simulink library "NeuroMuscularLibrary"  (R2019a)
settings: Solver=ode45  StartTime=0.0  StopTime=10.0  RelTol=1e-3  EnableMultiTasking=on
undefined symbols (not defined in the file): a2loptHAB, a2loptHAD, a2loptHAMsw, a2loptRFsw, ankle_height, aRefHAB, aRefHAD, aRefHAMsw, aRefRFsw, c, c_jointstop, deltaLegAngleThr, DeltaThRef, eref, Fmax, FmaxGLU, footBallToAnkleDist, footBallToCGDist, footBallToCGDist_y, footBallToHeelDist, footCenterlineToBall, footCenterlineToHeel, footInertia, footLength, footMass, FT, FT_GLU, GainDphiHATGLUst, GainDphiHATHABst, GainDphiHATHADst, GainDphiHATHFLst, GainFGASst, GainFGLUst, GainFHABst, GainFHAMst, GainFSOLst, GainFSOLTAst, GainFVASst, GainLBFSHst, GainLBFSHVASst, GainLGLUsw, GainLHABsw, GainLHADsw, GainLHAMGLUsw, GainLHAMsw, GainLRFHFLsw, GainLTAst, GainLTAsw, GainLVASsw, GainPhiHATGLUst, GainPhiHATHABst, GainPhiHATHADst, GainPhiHATHFLst, GainSGLUcHFLst, GainSGLUHAMst, GainSHABcHABst, GainSHADcHADst, GainSHAMBFSHsw, GainSHAMcHFLst, GainSHAMGASsw ... (+175)
libraries: sm_lib x54, $bdroot x45, nesl_utility x39, simulink x24, simulink_extras x6, vrlib x5, dspsigops x4
(part 4 of 5)

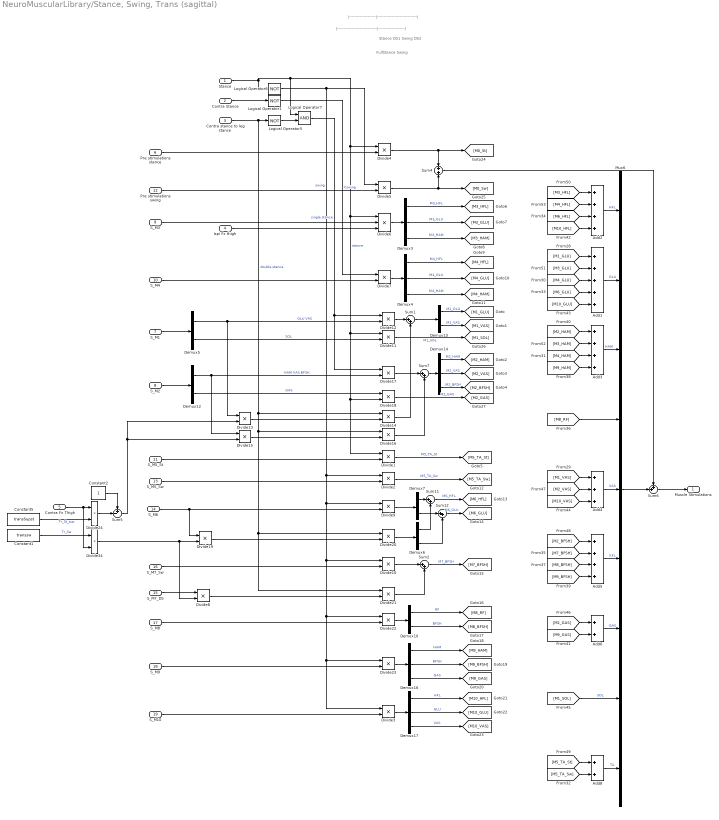
== system NeuroMuscularLibrary/Stance, Swing, Trans (sagittal) ==
  note: Stance DS1 Swing DS2
  note: FullStance Swing
  note: |------------------------------|--------------------|
  note: |--------------------|------------------------------|
  Stance : Inport
  Contra Stance : Inport  Port=2
  Contra stance to leg stance : Inport  Port=3
  Ispi Fx thigh : Inport  Port=4
  Contra Fx Thigh : Inport  Port=5
  Pre stimulations stance : Inport  Port=6
  S_M1 : Inport  Port=7
  S_M2 : Inport  Port=8
  S_M3 : Inport  Port=9
  S_M4 : Inport  Port=10
  S_M5_St : Inport  Port=11
  Pre stimulations swing : Inport  Port=12
  S_M5_Sw : Inport  Port=13
  S_M6 : Inport  Port=14
  S_M7_DS : Inport  Port=15
  S_M7_Sw : Inport  Port=16
  S_M8 : Inport  Port=17
  S_M9 : Inport  Port=18
  S_M10 : Inport  Port=19
  Add1 : Sum  Inputs=5
  Add2 : Sum  Inputs=4
  Add3 : Sum  Inputs=4
  Add4 : Sum  Inputs=3
  Add5 : Sum  Inputs=4
  Add6 : Sum  Inputs=2
  Add8 : Sum  Inputs=2
  Constant1 : Constant  Value=transsw
  Constant2 : Constant
  Constant5 : Constant  Value=transSupst
  Demux{6..7,10,13} (4 alike) : Demux  Outputs=2
  Demux12 : Demux  Outputs=[3 1]
  Demux{3..4,14,16..17} (5 alike) : Demux  Outputs=3
  Demux5 : Demux  Outputs=[2 1]
  Divide{1..5,7..24,34} (24 alike) : Product
  Divide6 : Product  Inputs=3
  Logical Operator1 : Logic  Operator=NOT  AllPortsSameDT=off  OutDataTypeStr=boolean
  Logical Operator5 : Logic  Operator=NOT  AllPortsSameDT=off  OutDataTypeStr=boolean
  Logical Operator6 : Logic  Operator=NOT  AllPortsSameDT=off  OutDataTypeStr=boolean
  Logical Operator7 : Logic  AllPortsSameDT=off  OutDataTypeStr=boolean
  Mux6 : Mux  Inputs=9
  Sum{1..2,7,11..12} (5 alike) : Sum  Inputs=|++  SaturateOnIntegerOverflow=on  InputSameDT=on  OutDataTypeStr=Inherit: Same as first input
  Sum4 : Sum  SaturateOnIntegerOverflow=on  InputSameDT=on  OutDataTypeStr=Inherit: Same as first input
  Sum5 : Sum  Inputs=+-|  SaturateOnIntegerOverflow=on  InputSameDT=on  OutDataTypeStr=Inherit: Same as first input
  Sum6 : Sum  Inputs=++|  SaturateOnIntegerOverflow=on  InputSameDT=on  OutDataTypeStr=Inherit: Same as first input
  Muscle Stimulations : Outport  OutputWhenDisabled=reset  InitialOutput=0  VectorParamsAs1DForOutWhenUnconnected=on
  wires:
  Stance/1 -> Logical Operator7/1, Divide4/1, Divide11/1, Divide18/2, Divide1/1, Divide6/1, Logical Operator6/1  "stance"
  Contra stance to leg stance/1 -> Logical Operator5/1, Divide14/1, Divide16/1, Divide20/1, Divide21/1  "double stance"
  Logical Operator5/1 -> Logical Operator7/2
  S_M4/1 -> Divide7/2
  Contra Stance/1 -> Logical Operator1/1
  Logical Operator1/1 -> Divide7/1  "Cswing"
  Constant5/1 -> Divide24/2  "Tr_St_sup"
  Divide24/1 -> Sum5/2
  Constant2/1 -> Sum5/1
  Contra Fx Thigh/1 -> Divide24/1, Divide34/2
  Demux4/1 -> [M4_HFL]  "M4_HFL"
  Add2/1 -> Mux6/1  "HFL"
  Add1/1 -> Mux6/2  "GLU"
  Demux4/2 -> [M4_GLU]  "M4_GLU"
  Add3/1 -> Mux6/3  "HAM"
  Demux4/3 -> [M4_HAM]  "M4_HAM"
  Add4/1 -> Mux6/5  "VAS"
  Add5/1 -> Mux6/6  "KFL"
  Add6/1 -> Mux6/7  "GAS"
  Add8/1 -> Mux6/9  "TA"
  Constant1/1 -> Divide34/1  "Tr_Sw"
  Divide7/1 -> Demux4/1
  Logical Operator7/1 -> Divide12/1, Divide17/1  "single stance"
  Divide34/1 -> Divide19/2, Divide8/2
  Logical Operator6/1 -> Divide5/1, Divide2/1, Divide9/1, Divide10/1, Divide3/1, Divide23/1, Divide22/1  "swing"
  Mux6/1 -> Sum6/2
  Sum6/1 -> Muscle Stimulations/1
  Sum4/1 -> Sum6/1
  Pre stimulations swing/1 -> Divide5/2
  Pre stimulations stance/1 -> Divide4/2
  Divide5/1 -> [M0_Sw], Sum4/2
  Divide4/1 -> Sum4/1, [M0_St]
  S_M1/1 -> Demux5/1
  S_M2/1 -> Demux12/1
  Demux5/1 -> Divide12/2, Divide13/1  "GLU VAS"
  Demux5/2 -> Divide11/2  "SOL"
  Divide12/1 -> Sum1/1
  Divide13/1 -> Divide14/2
  Divide14/1 -> Sum1/2
  Divide16/1 -> Sum7/2
  Divide15/1 -> Divide16/2
  Sum1/1 -> Demux13/1
  Demux13/1 -> [M1_GLU]  "M1_GLU"
  Demux13/2 -> [M1_VAS]  "M1_VAS"
  Demux12/1 -> Divide17/2, Divide15/1  "HAM VAS BFSH"
  Divide17/1 -> Sum7/1
  Sum7/1 -> Demux14/1
  Demux14/1 -> [M2_HAM]  "M2_HAM"
  Demux14/2 -> [M2_VAS]  "M2_VAS"
  Demux14/3 -> [M2_BFSH]  "M2_BFSH"
  Demux12/2 -> Divide18/1  "GAS"
  Divide18/1 -> [M2_GAS]  "M2_GAS"
  S_M5_St/1 -> Divide1/2
  Divide1/1 -> [M5_TA_St]  "M5_TA_St"
  Divide11/1 -> [M1_SOL]  "M1_SOL"
  S_M3/1 -> Divide6/2
  Ispi Fx thigh/1 -> Divide6/3
  Divide6/1 -> Demux3/1
  Demux3/1 -> [M3_HFL]  "M3_HFL"
  Demux3/2 -> [M3_GLU]  "M3_GLU"
  Demux3/3 -> [M3_HAM]  "M3_HAM"
  S_M5_Sw/1 -> Divide2/2
  Divide2/1 -> [M5_TA_Sw]  "M5_TA_Sw"
  S_M6/1 -> Divide9/2, Divide19/1
  Divide9/1 -> Demux7/1
  Demux7/2 -> Sum12/1
  Divide20/1 -> Demux6/1
  Demux6/1 -> Sum11/2
  Demux6/2 -> Sum12/2
  Demux7/1 -> Sum11/1
  Divide19/1 -> Divide20/2
  Sum11/1 -> [M6_HFL]  "M6_HFL"
  Sum12/1 -> [M6_GLU]  "M6_GLU"
  Divide10/1 -> Sum2/1
  Divide21/1 -> Sum2/2
  Sum5/1 -> Divide13/2, Divide15/2
  S_M7_Sw/1 -> Divide10/2
  Divide8/1 -> Divide21/2
  S_M7_DS/1 -> Divide8/1
  Sum2/1 -> [M7_BFSH]  "M7_BFSH"
  S_M8/1 -> Divide22/2
  Divide22/1 -> Demux10/1
  S_M9/1 -> Divide23/2
  Divide23/1 -> Demux16/1
  S_M10/1 -> Divide3/2
  Divide3/1 -> Demux17/1
  Demux10/2 -> [M8_BFSH]  "BFSH"
  Demux10/1 -> [M8_RF]  "RF"
  Demux16/1 -> [M9_HAM]  "HAM"
  Demux16/2 -> [M9_BFSH]  "BFSH"
  Demux16/3 -> [M9_GAS]  "GAS"
  Demux17/1 -> [M10_HFL]  "HFL"
  Demux17/2 -> [M10_GLU]  "GLU"
  Demux17/3 -> [M10_VAS]  "VAS"
  [M1_GLU] -> Add1/1
  [M3_GLU] -> Add1/2
  [M4_GLU] -> Add1/3
  [M6_GLU] -> Add1/4
  [M10_GLU] -> Add1/5
  [M1_VAS] -> Add4/1
  [M2_HAM] -> Add3/1
  [M2_VAS] -> Add4/2
  [M2_BFSH] -> Add5/1
  [M2_GAS] -> Add6/1
  [M3_HFL] -> Add2/1
  [M3_HAM] -> Add3/2
  [M4_HFL] -> Add2/2
  [M4_HAM] -> Add3/3
  [M5_TA_St] -> Add8/1
  [M5_TA_Sw] -> Add8/2
  [M6_HFL] -> Add2/3
  [M7_BFSH] -> Add5/2
  [M9_BFSH] -> Add5/4
  [M8_BFSH] -> Add5/3
  [M8_RF] -> Mux6/4
  [M9_HAM] -> Add3/4
  [M9_GAS] -> Add6/2
  [M10_HFL] -> Add2/4
  [M10_VAS] -> Add4/3
  [M1_SOL] -> Mux6/8  "SOL"

== system NeuroMuscularLibrary/Swing Phase (coronal) ==
  note: Swing Phase Control
  note: M6: swing hip
  Target Angle Coronal : Inport
  LceHAD : Inport  Port=2
  LceHAB : Inport  Port=3
  Enable : EnablePort  StatesWhenEnabling=reset  ZeroCross=off
  " 1" : Gain  Gain=a2loptHAB
  " 2" : Gain  Gain=a2loptHAD
  " 3" : Gain  Gain=GainLHABsw
  " 4" : Gain  Gain=GainLHADsw
  Constant1 : Constant
  Constant12 : Constant  Value=PreStimHADsw
  Constant15 : Constant  Value=PreStimHABsw
  Constant2 : Constant  Value=aRefHAB
  Constant3 : Constant  Value=aRefHAD
  Constant5 : Constant
  Mux : Mux  Inputs=2
  Mux1 : Mux  Inputs=2
  Sum1 : Sum  Inputs=-+|  SaturateOnIntegerOverflow=on  InputSameDT=on  OutDataTypeStr=Inherit: Same as first input
  Sum10 : Sum  Inputs=++|  SaturateOnIntegerOverflow=on  InputSameDT=on  OutDataTypeStr=Inherit: Same as first input
  Sum13 : Sum  Inputs=|-+  SaturateOnIntegerOverflow=on  InputSameDT=on  OutDataTypeStr=Inherit: Same as first input
  Sum2 : Sum  Inputs=-+|  SaturateOnIntegerOverflow=on  InputSameDT=on  OutDataTypeStr=Inherit: Same as first input
  Sum3 : Sum  Inputs=+-|  SaturateOnIntegerOverflow=on  InputSameDT=on  OutDataTypeStr=Inherit: Same as first input
  Sum4 : Sum  Inputs=+-|  SaturateOnIntegerOverflow=on  InputSameDT=on  OutDataTypeStr=Inherit: Same as first input
  positive half1 : Saturate  UpperLimit=inf  LowerLimit=0  ZeroCross=off
  positive half2 : Saturate  UpperLimit=inf  LowerLimit=0  ZeroCross=off
  S_0_Sw : Outport  OutputWhenDisabled=reset  InitialOutput=0  VectorParamsAs1DForOutWhenUnconnected=on
  S_M6 [HAB HAD] : Outport  Port=2  OutputWhenDisabled=reset  InitialOutput=0  VectorParamsAs1DForOutWhenUnconnected=on
  wires:
  Mux/1 -> S_0_Sw/1
  Constant5/1 -> Sum10/1
  Sum13/1 -> " 1"/1
  " 1"/1 -> Sum10/2
  Sum10/1 -> Sum1/1  "lceOffHAB"
  Sum1/1 -> positive half2/1
  positive half2/1 -> " 3"/1
  Constant1/1 -> Sum3/1
  Target Angle Coronal/1 -> Sum13/2, Sum4/1
  Sum4/1 -> " 2"/1
  " 2"/1 -> Sum3/2
  Sum3/1 -> Sum2/1  "lceOffHAD"
  Sum2/1 -> positive half1/1
  positive half1/1 -> " 4"/1
  LceHAB/1 -> Sum1/2
  LceHAD/1 -> Sum2/2
  " 3"/1 -> Mux1/1  "HAB"
  " 4"/1 -> Mux1/2  "HAD"
  Mux1/1 -> S_M6 [HAB HAD]/1
  Constant15/1 -> Mux/1
  Constant12/1 -> Mux/2
  Constant2/1 -> Sum13/1
  Constant3/1 -> Sum4/2

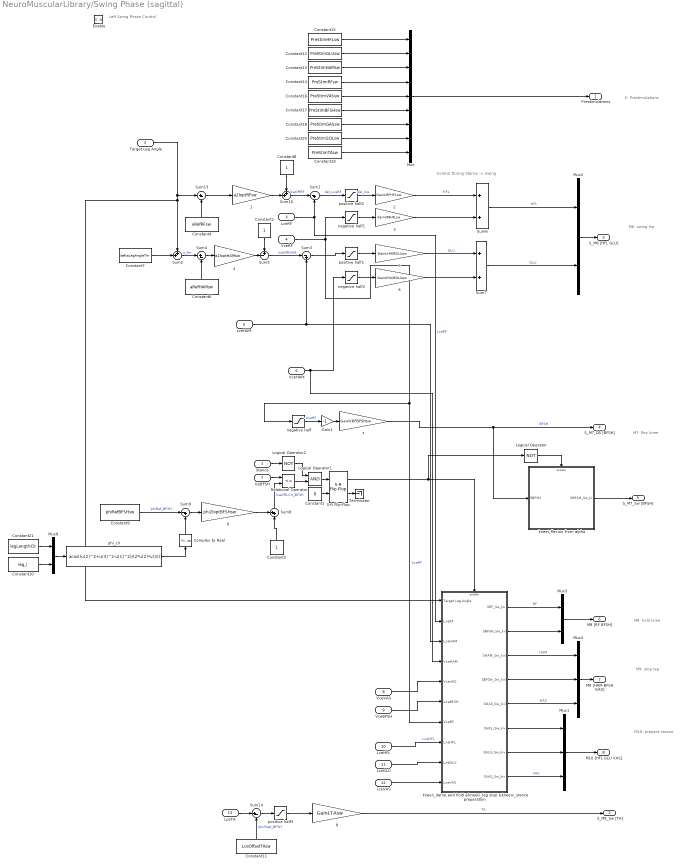
== system NeuroMuscularLibrary/Swing Phase (sagittal) ==
  note: Left Swing Phase Control
  note: Control During Stance -> Swing
  note: 0: Prestimulations
  note: M6: swing hip
  note: M7: flex knee
  note: M8: hold knee
  note: M9: stop leg
  note: M10: prepare stance
  Stance : Inport
  "Target Leg Angle " : Inport  Port=2
  LceRF : Inport  Port=3
  VceRF : Inport  Port=4
  LceHAM : Inport  Port=5
  VceHAM : Inport  Port=6
  lceBFSH : Inport  Port=7
  VceVAS : Inport  Port=8
  VceBFSH : Inport  Port=9
  LceHFL : Inport  Port=10
  LceGLU : Inport  Port=11
  LceVAS : Inport  Port=12
  LceTA : Inport  Port=13
  Enable : EnablePort  StatesWhenEnabling=reset  ZeroCross=off
  " 1" : Gain  Gain=a2loptRFsw
  " 2" : Gain  Gain=GainLRFHFLsw
  " 3" : Gain  Gain=GainVRFHFLsw
  " 4" : Gain  Gain=a2loptHAMsw
  " 5" : Gain  Gain=GainLHAMGLUsw
  " 6" : Gain  Gain=GainVHAMGLUsw
  " 7" : Gain  Gain=GainVRFBFSHsw
  " 8" : Gain  Gain=GainLTAsw
  " 9" : Gain  Gain=phi2loptBFSHsw
  Complex to Real : ComplexToRealImag  Output=Real
  Constant1 : Constant  Value=0  OutDataTypeStr=boolean
  Constant10 : Constant  Value=leg_l
  Constant11 : Constant  Value=LceOffsetTAsw
  Constant12 : Constant  Value=PreStimGLUsw
  Constant13 : Constant  Value=PreStimHAMsw
  Constant14 : Constant  Value=PreStimRFsw
  Constant15 : Constant  Value=PreStimHFLsw
  Constant16 : Constant  Value=PreStimVASsw
  Constant17 : Constant  Value=PreStimBFSHsw
  Constant18 : Constant  Value=PreStimGASsw
  Constant19 : Constant  Value=PreStimTAsw
  Constant2 : Constant
  Constant20 : Constant  Value=PreStimSOLsw
  Constant21 : Constant  Value=legLengthClr
  Constant3 : Constant
  Constant4 : Constant  Value=aRefRFsw
  Constant6 : Constant  Value=aRefHAMsw
  Constant7 : Constant  Value=deltaLegAngleThr
  Constant8 : Constant
  Constant9 : Constant  Value=phiRefBFSHsw
  Gain1 : Gain  Gain=-1
  Logical Operator : Logic  Operator=NOT  AllPortsSameDT=off  OutDataTypeStr=boolean
  Logical Operator1 : Logic  AllPortsSameDT=off  OutDataTypeStr=boolean
  Logical Operator2 : Logic  Operator=NOT  AllPortsSameDT=off  OutDataTypeStr=boolean
  Mux : Mux  Inputs=9
  Mux1 : Mux  Inputs=3
  Mux2 : Mux  Inputs=2
  Mux3 : Mux  Inputs=2
  Mux4 : Mux  Inputs=3
  Mux8 : Mux  Inputs=2
  Relational Operator : RelationalOperator  Operator=<=  OutDataTypeStr=boolean  ZeroCross=off  RndMeth=Nearest
  S-R Flip-Flop : simulink_extras/Flip Flops/S-R Flip-Flop  initial_condition=0
  Sum1 : Sum  Inputs=|-+  SaturateOnIntegerOverflow=on  InputSameDT=on  OutDataTypeStr=Inherit: Same as first input
  Sum10 : Sum  Inputs=++|  SaturateOnIntegerOverflow=on  InputSameDT=on  OutDataTypeStr=Inherit: Same as first input
  Sum13 : Sum  Inputs=|+-  SaturateOnIntegerOverflow=on  InputSameDT=on  OutDataTypeStr=Inherit: Same as first input
  Sum14 : Sum  Inputs=|+-  SaturateOnIntegerOverflow=on  InputSameDT=on  OutDataTypeStr=Inherit: Same as first input
  Sum2 : Sum  Inputs=++|  SaturateOnIntegerOverflow=on  InputSameDT=on  OutDataTypeStr=Inherit: Same as first input
  Sum3 : Sum  Inputs=|-+  SaturateOnIntegerOverflow=on  InputSameDT=on  OutDataTypeStr=Inherit: Same as first input
  Sum4 : Sum  Inputs=|+-  SaturateOnIntegerOverflow=on  InputSameDT=on  OutDataTypeStr=Inherit: Same as first input
  Sum5 : Sum  Inputs=+-|  SaturateOnIntegerOverflow=on  InputSameDT=on  OutDataTypeStr=Inherit: Same as first input
  Sum6 : Sum  SaturateOnIntegerOverflow=on  InputSameDT=on  OutDataTypeStr=Inherit: Same as first input
  Sum7 : Sum  SaturateOnIntegerOverflow=on  InputSameDT=on  OutDataTypeStr=Inherit: Same as first input
  Sum8 : Sum  Inputs=++|  SaturateOnIntegerOverflow=on  InputSameDT=on  OutDataTypeStr=Inherit: Same as first input
  Sum9 : Sum  Inputs=|-+  SaturateOnIntegerOverflow=on  InputSameDT=on  OutDataTypeStr=Inherit: Same as first input
  Terminator : Terminator
  kneei_flexion from alpha : Subsystem  TreatAsAtomicUnit=on
  kneeii_damp and hold &kneeiii_leg stop &kneeiv_stance preparation : Subsystem  TreatAsAtomicUnit=on
  negative half : Saturate  UpperLimit=0  LowerLimit=-inf  ZeroCross=off
  negative half1 : Saturate  UpperLimit=0  LowerLimit=-inf  ZeroCross=off
  negative half2 : Saturate  UpperLimit=0  LowerLimit=-inf  ZeroCross=off
  phi_clr : Fcn  Expr=acos((u(2)^2+u(3)^2-u(1)^2)/(2*u(2)*u(3)))
  positive half1 : Saturate  UpperLimit=inf  LowerLimit=0  ZeroCross=off
  positive half2 : Saturate  UpperLimit=inf  LowerLimit=0  ZeroCross=off
  positive half3 : Saturate  UpperLimit=inf  LowerLimit=0  ZeroCross=off
  Prestimulations : Outport  OutputWhenDisabled=reset  InitialOutput=0  VectorParamsAs1DForOutWhenUnconnected=on
  S_M5_Sw [TA] : Outport  Port=2  OutputWhenDisabled=reset  InitialOutput=0  VectorParamsAs1DForOutWhenUnconnected=on
  S_M6 [HFL GLU] : Outport  Port=3  OutputWhenDisabled=reset  InitialOutput=0  VectorParamsAs1DForOutWhenUnconnected=on
  S_M7_DS [BFSH] : Outport  Port=4  OutputWhenDisabled=reset  InitialOutput=0  VectorParamsAs1DForOutWhenUnconnected=on
  S_M7_Sw [BFSH] : Outport  Port=5  OutputWhenDisabled=reset  InitialOutput=0  VectorParamsAs1DForOutWhenUnconnected=on
  M8 [RF BFSH] : Outport  Port=6  OutputWhenDisabled=reset  InitialOutput=0  VectorParamsAs1DForOutWhenUnconnected=on
  M9 [HAM BFSH GAS] : Outport  Port=7  OutputWhenDisabled=reset  InitialOutput=0  VectorParamsAs1DForOutWhenUnconnected=on
  M10 [HFL GLU VAS] : Outport  Port=8  OutputWhenDisabled=reset  InitialOutput=0  VectorParamsAs1DForOutWhenUnconnected=on
  wires:
  "Target Leg Angle "/1 -> kneeii_damp and hold &kneeiii_leg stop &kneeiv_stance preparation/1(Target Leg Angle), Sum2/1, Sum13/1
  Sum13/1 -> " 1"/1
  " 1"/1 -> Sum10/2
  Sum1/1 -> positive half2/1  "del_LceRF"
  positive half2/1 -> " 2"/1  "del_lce"
  Sum2/1 -> Sum4/1  "a_thr"
  Constant2/1 -> Sum5/1
  " 4"/1 -> Sum5/2
  Sum3/1 -> positive half1/1
  positive half1/1 -> " 5"/1
  Sum5/1 -> Sum3/1  "lceOffHAM"
  LceHAM/1 -> Sum3/2, kneeii_damp and hold &kneeiii_leg stop &kneeiv_stance preparation/3(LceHAM)
  Gain1/1 -> " 7"/1
  negative half/1 -> Gain1/1  "-VceRF"
  " 7"/1 -> kneei_flexion from alpha/1(SBFSH), S_M7_DS [BFSH]/1  "BFSH"
  Constant1/1 -> S-R Flip-Flop/2
  S-R Flip-Flop/2 -> Terminator/1
  S-R Flip-Flop/1 -> Logical Operator/1, kneeii_damp and hold &kneeiii_leg stop &kneeiv_stance preparation/Enable
  Logical Operator/1 -> kneei_flexion from alpha/Enable
  lceBFSH/1 -> Relational Operator/1
  Mux8/1 -> phi_clr/1
  Constant21/1 -> Mux8/1
  Constant10/1 -> Mux8/2
  Sum9/1 -> " 9"/1
  Constant9/1 -> Sum9/1  "phiRef_BFSH"
  phi_clr/1 -> Complex to Real/1
  Constant3/1 -> Sum8/2
  " 9"/1 -> Sum8/1
  Sum8/1 -> Relational Operator/2  "lceOffLClr_BFSH"
  VceBFSH/1 -> kneeii_damp and hold &kneeiii_leg stop &kneeiv_stance preparation/6(VceBFSH)
  LceHFL/1 -> kneeii_damp and hold &kneeiii_leg stop &kneeiv_stance preparation/8(LceHFL)  "LceHFL"
  LceGLU/1 -> kneeii_damp and hold &kneeiii_leg stop &kneeiv_stance preparation/9(LceGLU)
  LceVAS/1 -> kneeii_damp and hold &kneeiii_leg stop &kneeiv_stance preparation/10(LceVAS)
  kneeii_damp and hold &kneeiii_leg stop &kneeiv_stance preparation/6(SHFL_Sw_kiv) -> Mux1/1
  kneeii_damp and hold &kneeiii_leg stop &kneeiv_stance preparation/7(SGLU_Sw_kiv) -> Mux1/2
  kneei_flexion from alpha/1(SBFSH_Sw_ki) -> S_M7_Sw [BFSH]/1
  kneeii_damp and hold &kneeiii_leg stop &kneeiv_stance preparation/2(SBFSH_Sw_kii) -> Mux3/2
  kneeii_damp and hold &kneeiii_leg stop &kneeiv_stance preparation/4(SBFSH_Sw_kiii) -> Mux4/2
  Sum14/1 -> positive half3/1
  LceTA/1 -> Sum14/1
  positive half3/1 -> " 8"/1
  Logical Operator1/1 -> S-R Flip-Flop/1
  Relational Operator/1 -> Logical Operator1/2
  Stance/1 -> Logical Operator2/1
  Logical Operator2/1 -> Logical Operator1/1
  kneeii_damp and hold &kneeiii_leg stop &kneeiv_stance preparation/3(SHAM_Sw_kiii) -> Mux4/1  "HAM"
  kneeii_damp and hold &kneeiii_leg stop &kneeiv_stance preparation/1(SRF_Sw_kii) -> Mux3/1  "RF"
  kneeii_damp and hold &kneeiii_leg stop &kneeiv_stance preparation/8(SVAS_Sw_kiv) -> Mux1/3  "VAS"
  " 8"/1 -> S_M5_Sw [TA]/1  "TA"
  kneeii_damp and hold &kneeiii_leg stop &kneeiv_stance preparation/5(SGAS_Sw_kiii) -> Mux4/3  "GAS"
  Mux2/1 -> S_M6 [HFL GLU]/1
  Mux3/1 -> M8 [RF BFSH]/1
  Mux4/1 -> M9 [HAM BFSH GAS]/1
  Mux1/1 -> M10 [HFL GLU VAS]/1
  LceRF/1 -> kneeii_damp and hold &kneeiii_leg stop &kneeiv_stance preparation/2(LceRF), Sum1/2  "LceRF"
  VceVAS/1 -> kneeii_damp and hold &kneeiii_leg stop &kneeiv_stance preparation/5(VceVAS)
  VceRF/1 -> kneeii_damp and hold &kneeiii_leg stop &kneeiv_stance preparation/7(VceRF), negative half/1, negative half1/1  "VceRF"
  VceHAM/1 -> kneeii_damp and hold &kneeiii_leg stop &kneeiv_stance preparation/4(VceHAM), negative half2/1
  " 2"/1 -> Sum6/1  "HFL"
  " 3"/1 -> Sum6/2
  Sum6/1 -> Mux2/1  "HFL"
  negative half1/1 -> " 3"/1
  negative half2/1 -> " 6"/1
  " 5"/1 -> Sum7/1  "GLU"
  Sum7/1 -> Mux2/2  "GLU"
  " 6"/1 -> Sum7/2
  Constant4/1 -> Sum13/2
  Constant7/1 -> Sum2/2
  Constant6/1 -> Sum4/2
  Constant8/1 -> Sum10/1
  Sum10/1 -> Sum1/1  "lceOffRF"
  Sum4/1 -> " 4"/1
  Constant11/1 -> Sum14/2  "phi2lopt_BFSH"
  Constant14/1 -> Mux/4
  Constant12/1 -> Mux/2
  Mux/1 -> Prestimulations/1
  Constant19/1 -> Mux/9
  Constant17/1 -> Mux/6
  Constant18/1 -> Mux/7
  Constant15/1 -> Mux/1
  Constant13/1 -> Mux/3
  Constant16/1 -> Mux/5
  Constant20/1 -> Mux/8
  Complex to Real/1 -> Sum9/2

== system NeuroMuscularLibrary/TA Link ==
  note: TA Attachment
  Ankle angle  [rad] : Inport
  Constant : Constant  Value=lslackTA+loptTA
  Constant3 : Constant  Value=phimaxTA
  Constant5 : Constant  Value=phirefTA
  Demux1 : Demux  Outputs=2
  Gain2 : Gain  Gain=rTAmax
  Gain3 : Gain  Gain=phiScaleTA
  Gain8 : Gain  Gain=phiScaleTA
  Gain9 : Gain  Gain=rhoTA/phiScaleTA
  Mux1 : Mux  Inputs=2
  Sum4 : Sum  Inputs=-+
  Sum5 : Sum  Inputs=|++
  Sum6 : Sum  Inputs=|+-
  Sum7 : Sum  Inputs=-+|
  length change term : Trigonometry
  offset correction term : Trigonometry
  variable lever term : Trigonometry  Operator=cos
  lmtc [m] : Outport  VectorParamsAs1DForOutWhenUnconnected=on
  lever [m] : Outport  Port=2  VectorParamsAs1DForOutWhenUnconnected=on
  wires:
  Sum7/1 -> Gain3/1
  Sum6/1 -> Gain8/1
  length change term/1 -> Sum4/2
  variable lever term/1 -> Mux1/2
  Gain8/1 -> offset correction term/1
  Sum4/1 -> Mux1/1
  Constant5/1 -> Sum6/1
  Mux1/1 -> Gain2/1
  Gain9/1 -> Sum5/2
  Demux1/2 -> lever [m]/1
  Sum5/1 -> lmtc [m]/1
  Constant3/1 -> Sum7/1, Sum6/2
  offset correction term/1 -> Sum4/1
  Gain3/1 -> variable lever term/1, length change term/1
  Gain2/1 -> Demux1/1
  Demux1/1 -> Gain9/1
  Constant/1 -> Sum5/1
  Ankle angle  [rad]/1 -> Sum7/2

== system NeuroMuscularLibrary/Target leg angle calculator ==
  note: positive for left, negative for right
  Saggital d,v : Inport
  Coronal d,v : Inport  Port=2
  HATy : Inport  Port=3
  HATyInt : Inport  Port=4
  " 1" : Gain  Gain=simbiconGainV
  " 2" : Gain  Gain=simbiconGainV_C
  " 3" : Gain  Gain=simbiconGainD
  " 4" : Gain  Gain=simbiconGainD_C
  " 5" : Gain  Gain=headingGain
  " 6" : Gain  Gain=headingIntGain
  Add : Sum  Inputs=+--
  Add1 : Sum  Inputs=+++++
  Constant2 : Constant  Value=simbiconLegAngle0
  Constant7 : Constant  Value=simbiconLegAngle0_C
  Demux : Demux  Outputs=2
  Demux1 : Demux  Outputs=2
  "Saggital Target leg angle " : Outport  VectorParamsAs1DForOutWhenUnconnected=on
  "Coronal Target leg angle " : Outport  Port=2  VectorParamsAs1DForOutWhenUnconnected=on
  wires:
  Saggital d,v/1 -> Demux/1
  Coronal d,v/1 -> Demux1/1
  Demux/1 -> " 3"/1  "d"
  Demux/2 -> " 1"/1  "v"
  Demux1/1 -> " 4"/1  "d"
  Demux1/2 -> " 2"/1  "v"
  " 1"/1 -> Add/3
  " 3"/1 -> Add/2
  Constant2/1 -> Add/1
  Constant7/1 -> Add1/1
  " 4"/1 -> Add1/2
  " 2"/1 -> Add1/3
  Add/1 -> "Saggital Target leg angle "/1
  HATy/1 -> " 5"/1
  " 5"/1 -> Add1/4
  Add1/1 -> "Coronal Target leg angle "/1
  " 6"/1 -> Add1/5
  HATyInt/1 -> " 6"/1

== system NeuroMuscularLibrary/Thigh Sensor Sheet ==
  note: Inner Segment Pressure Sheet
  Gain3 : Gain  Gain=k_pressure
  Gain4 : Gain  Gain=1/v_max_pressure
  Mux1 : Mux  Inputs=2
  PS-Simulink Converter : nesl_utility/PS-Simulink Converter  PhysicalDomain=network_engine_domain  SubClassName=ps_output  LeftPortType=input  RightPortType=output  PseudoPeriodic=off  Frequencies=[]  Unit=m/s  AffineConversion=off
  PS-Simulink Converter1 : nesl_utility/PS-Simulink Converter  PhysicalDomain=network_engine_domain  SubClassName=ps_output  LeftPortType=input  RightPortType=output  PseudoPeriodic=off  Frequencies=[]  Unit=m  AffineConversion=off
  Pressure Sheet Reaction Force : Fcn  Expr=-u(1) * (1+sgn(u(1))*u(2))
  Prismatic Joint : sm_lib/Joints/Prismatic Joint  SenseConstraintForce=off  SenseConstraintForceX=off  SenseConstraintForceY=off  SenseConstraintForceZ=off  SenseConstraintTorque=off  SenseConstraintTorqueX=off  SenseConstraintTorqueY=off  SenseConstraintTorqueZ=off  SenseTotalForce=off  SenseTotalForceX=off  SenseTotalForceY=off  SenseTotalForceZ=off  SenseTotalTorque=off  SenseTotalTorqueX=off  SenseTotalTorqueY=off  SenseTotalTorqueZ=off  CompositeWrenchDir=FollowerOnBase  CompositeWrenchFrame=BaseFrame  EquilibriumPosition=0  EquilibriumPositionUnits=m  SpringStiffness=0  SpringStiffnessUnits=N/m  DampingCoefficient=0  DampingCoefficientUnits=N/(m/s)  TorqueActuationMode=InputTorque  MotionActuationMode=ComputedMotion  SensePosition=on  SenseVelocity=on  SenseAcceleration=off  SenseTorqueForce=off  SenseLowerLimitTorqueForce=off  SenseUpperLimitTorqueForce=off  LowerLimitSpecify=off  LowerLimitBound=-1  LowerLimitBoundUnits=m  LowerLimitStiffness=1e6  LowerLimitStiffnessUnits=N/m  LowerLimitDamping=1e3  LowerLimitDampingUnits=N/(m/s)  LowerLimitTransitionRegionWidth=1e-4  LowerLimitTransitionRegionWidthUnits=m  UpperLimitSpecify=off  UpperLimitBound=1  UpperLimitBoundUnits=m  UpperLimitStiffness=1e6  UpperLimitStiffnessUnits=N/m  UpperLimitDamping=1e3  UpperLimitDampingUnits=N/(m/s)  UpperLimitTransitionRegionWidth=1e-4  UpperLimitTransitionRegionWidthUnits=m  PositionTargetSpecify=on  PositionTargetPriority=High  PositionTargetValue=0  PositionTargetValueUnits=m  VelocityTargetSpecify=on  VelocityTargetPriority=High  VelocityTargetValue=0  VelocityTargetValueUnits=m/s
  Rigid Transform : sm_lib/Frames and Transforms/Rigid Transform  TranslationMethod=None  TranslationStandardOffset=0  TranslationLengthUnit=m  TranslationStandardAxis=+Z  TranslationCartesianOffset=[0 0 0]  TranslationROffset=0  TranslationROffsetUnits=m  TranslationZOffset=0  TranslationZOffsetUnits=m  TranslationThetaOffset=0  TranslationThetaOffsetUnits=deg  RotationMethod=AlignedAxes  RotationAngleUnits=deg  RotationStandardAxis=+Z  RotationAngle=0.0  RotationArbitraryAxis=[0 0 1]  FollAlignAxisA=+Z  BaseAlignAxisA=+X  FollAlignAxisB=+Y  BaseAlignAxisB=+Y  RotationSequenceAxes=FollowerAxes  RotationSequence=XYX  RotationSequenceAngles=[0 0 0]  RotationSequenceAnglesUnits=deg  RotationMatrix=[1 0 0; 0 1 0; 0 0 1]
  Rigid Transform1 : sm_lib/Frames and Transforms/Rigid Transform  TranslationMethod=None  TranslationStandardOffset=0  TranslationLengthUnit=m  TranslationStandardAxis=+Z  TranslationCartesianOffset=[0 0 0]  TranslationROffset=0  TranslationROffsetUnits=m  TranslationZOffset=0  TranslationZOffsetUnits=m  TranslationThetaOffset=0  TranslationThetaOffsetUnits=deg  RotationMethod=AlignedAxes  RotationAngleUnits=deg  RotationStandardAxis=+Z  RotationAngle=0.0  RotationArbitraryAxis=[0 0 1]  FollAlignAxisA=+X  BaseAlignAxisA=+Z  FollAlignAxisB=+Y  BaseAlignAxisB=+Y  RotationSequenceAxes=FollowerAxes  RotationSequence=XYX  RotationSequenceAngles=[0 0 0]  RotationSequenceAnglesUnits=deg  RotationMatrix=[1 0 0; 0 1 0; 0 0 1]
  Simulink-PS Converter : nesl_utility/Simulink-PS Converter  PhysicalDomain=network_engine_domain  SubClassName=ps_input  LeftPortType=input  RightPortType=output  PseudoPeriodic=off  Frequencies=[]  NoiseDistribution=none  NoiseParameters=[]  Unit=N  AffineConversion=off  FilteringAndDerivatives=provide  SimscapeFilterOrder=1  InputFilterTimeConstant=0.001  UdotUserProvided=0
  B : PMIOPort  Tag=PMCPort  Side=Left
  F : PMIOPort  Tag=PMCPort  Port=2  Side=Right
  dx : Outport  VectorParamsAs1DForOutWhenUnconnected=on
  wires:
  PS-Simulink Converter1/1 -> Gain3/1, dx/1
  PS-Simulink Converter/1 -> Gain4/1
  Mux1/1 -> Pressure Sheet Reaction Force/1
  Gain3/1 -> Mux1/1
  Gain4/1 -> Mux1/2
  Pressure Sheet Reaction Force/1 -> Simulink-PS Converter/1
  connections:
  Rigid Transform/LConn1 -- B/RConn1
  Rigid Transform1/LConn1 -- Prismatic Joint/RConn1
  Prismatic Joint/LConn2 -- Simulink-PS Converter/RConn1
  PS-Simulink Converter1/LConn1 -- Prismatic Joint/RConn2
  PS-Simulink Converter/LConn1 -- Prismatic Joint/RConn3
  Prismatic Joint/LConn1 -- Rigid Transform/RConn1
  F/RConn1 -- Rigid Transform1/RConn1

== system NeuroMuscularLibrary/Thigh high ==
  Inertia : sm_lib/Body Elements/Inertia  InertiaType=Custom  Mass=thighMass*(1-relThighSensorPos)  MassUnits=kg  CenterOfMass=[0 0 0]  CenterOfMassUnits=m  MomentsOfInertia=thighInertiaHigh  MomentsOfInertiaUnits=kg*m^2  ProductsOfInertia=[0 0 0]  ProductsOfInertiaUnits=kg*m^2  GraphicType=None  MarkerShape=Inertia  MarkerSize=20  GraphicVisPropType=SimpleVisualProperties  GraphicDiffuseColor=[0.5 0.5 0.5]  GraphicSpecularColor=[0.5 0.5 0.5 1.0]  GraphicAmbientColor=[0.15 0.15 0.15 1.0]  GraphicEmissiveColor=[0.0 0.0 0.0 1.0]  GraphicShininess=75  GraphicOpacity=1.0
  Sensor sheet to hip : sm_lib/Frames and Transforms/Rigid Transform  TranslationMethod=Cartesian  TranslationStandardOffset=0  TranslationLengthUnit=m  TranslationStandardAxis=+Z  TranslationCartesianOffset=[-thighLength*(1-relThighSensorPos) 0 0]  TranslationROffset=0  TranslationROffsetUnits=m  TranslationZOffset=0  TranslationZOffsetUnits=m  TranslationThetaOffset=0  TranslationThetaOffsetUnits=deg  RotationMethod=AlignedAxes  RotationAngleUnits=deg  RotationStandardAxis=+Z  RotationAngle=0.0  RotationArbitraryAxis=[0 0 1]  FollAlignAxisA=+X  BaseAlignAxisA=+Z  FollAlignAxisB=+Y  BaseAlignAxisB=-Y  RotationSequenceAxes=FollowerAxes  RotationSequence=XYX  RotationSequenceAngles=[0 0 0]  RotationSequenceAnglesUnits=deg  RotationMatrix=[1 0 0; 0 1 0; 0 0 1]
  To CG : sm_lib/Frames and Transforms/Rigid Transform  TranslationMethod=Cartesian  TranslationStandardOffset=0  TranslationLengthUnit=m  TranslationStandardAxis=+Z  TranslationCartesianOffset=[-thighKneeToCG*(1-relThighSensorPos) 0 0]  TranslationROffset=0  TranslationROffsetUnits=m  TranslationZOffset=0  TranslationZOffsetUnits=m  TranslationThetaOffset=0  TranslationThetaOffsetUnits=deg  RotationMethod=AlignedAxes  RotationAngleUnits=deg  RotationStandardAxis=+Z  RotationAngle=0.0  RotationArbitraryAxis=[0 0 1]  FollAlignAxisA=+X  BaseAlignAxisA=+Y  FollAlignAxisB=+Z  BaseAlignAxisB=-X  RotationSequenceAxes=FollowerAxes  RotationSequence=XYX  RotationSequenceAngles=[0 0 0]  RotationSequenceAnglesUnits=deg  RotationMatrix=[1 0 0; 0 1 0; 0 0 1]
  sensor sheet : PMIOPort  Side=Right
  hip : PMIOPort  Port=2  Side=Left
  connections:
  sensor sheet/RConn1 -- Sensor sheet to hip/LConn1 -- To CG/LConn1
  To CG/RConn1 -- Inertia/RConn1
  hip/RConn1 -- Sensor sheet to hip/RConn1

== system NeuroMuscularLibrary/Thigh low ==
  Cylindrical Solid : sm_lib/Body Elements/Solid  InertiaType=CalculateFromGeometry  Mass=0  MassUnits=kg  CenterOfMass=[0 0 0]  CenterOfMassUnits=m  MomentsOfInertia=[1 1 1]  MomentsOfInertiaUnits=kg*m^2  ProductsOfInertia=[0 0 0]  ProductsOfInertiaUnits=kg*m^2  BasedOnType=Mass  Density=0  DensityUnits=kg/m^3  DoExposeReferenceFrame=on  SerializedFrames=<Frames/>  GraphicType=FromGeometry  MarkerShape=Sphere  MarkerSize=10  GraphicVisPropType=SimpleVisualProperties  GraphicDiffuseColor=[0.5 0.5 0.5]  GraphicSpecularColor=[0.5 0.5 0.5 1.0]  GraphicAmbientColor=[0.15 0.15 0.15 1.0]  GraphicEmissiveColor=[0.0 0.0 0.0 1.0]  GraphicShininess=75  GraphicOpacity=1.0  GeometryShape=Cylinder  RectangleSize=[1 1]  RectangleSizeUnits=m  BrickDimensions=[1 1 1]  BrickDimensionUnits=m  CylinderRadius=.075  CylinderRadiusUnits=m  CylinderLength=thighLength  CylinderLengthUnits=m  SphereRadius=1  SphereRadiusUnits=m  EllipsoidRadii=[1 1 1]  EllipsoidRadiiUnits=m  ExtrusionCrossSection=[1 1; -1 1; -1 -1; 1 -1]  ExtrusionCrossSectionUnits=m  ExtrusionLength=1  ExtrusionLengthUnits=m  PolygonNumSides=3  PolygonOuterRadius=1  PolygonOuterRadiusUnits=m  ExtGeomFileType=STEP  ExtGeomFileUnits=m  RevolutionCrossSection=[1 1; 1 -1; 2 -1; 2 1]  RevolutionCrossSectionUnits=m  RevolutionExtent=Full  RevolutionAngle=180  RevolutionAngleUnits=deg
  Inertia : sm_lib/Body Elements/Inertia  InertiaType=Custom  Mass=thighMass*relThighSensorPos  MassUnits=kg  CenterOfMass=[0 0 0]  CenterOfMassUnits=m  MomentsOfInertia=thighInertiaLow  MomentsOfInertiaUnits=kg*m^2  ProductsOfInertia=[0 0 0]  ProductsOfInertiaUnits=kg*m^2  GraphicType=None  MarkerShape=Inertia  MarkerSize=20  GraphicVisPropType=SimpleVisualProperties  GraphicDiffuseColor=[0.5 0.5 0.5]  GraphicSpecularColor=[0.5 0.5 0.5 1.0]  GraphicAmbientColor=[0.15 0.15 0.15 1.0]  GraphicEmissiveColor=[0.0 0.0 0.0 1.0]  GraphicShininess=75  GraphicOpacity=1.0
  Knee to Sensorsheet : sm_lib/Frames and Transforms/Rigid Transform  TranslationMethod=Cartesian  TranslationStandardOffset=0  TranslationLengthUnit=m  TranslationStandardAxis=+Z  TranslationCartesianOffset=[-thighLength*relThighSensorPos 0 0]  TranslationROffset=0  TranslationROffsetUnits=m  TranslationZOffset=0  TranslationZOffsetUnits=m  TranslationThetaOffset=0  TranslationThetaOffsetUnits=deg  RotationMethod=None  RotationAngleUnits=deg  RotationStandardAxis=+Z  RotationAngle=0.0  RotationArbitraryAxis=[0 0 1]  FollAlignAxisA=+X  BaseAlignAxisA=+Y  FollAlignAxisB=+Y  BaseAlignAxisB=+Z  RotationSequenceAxes=FollowerAxes  RotationSequence=XYX  RotationSequenceAngles=[0 0 0]  RotationSequenceAnglesUnits=deg  RotationMatrix=[1 0 0; 0 1 0; 0 0 1]
  To CG : sm_lib/Frames and Transforms/Rigid Transform  TranslationMethod=Cartesian  TranslationStandardOffset=0  TranslationLengthUnit=m  TranslationStandardAxis=+Z  TranslationCartesianOffset=[-thighKneeToCG*relThighSensorPos 0 0]  TranslationROffset=0  TranslationROffsetUnits=m  TranslationZOffset=0  TranslationZOffsetUnits=m  TranslationThetaOffset=0  TranslationThetaOffsetUnits=deg  RotationMethod=AlignedAxes  RotationAngleUnits=deg  RotationStandardAxis=+Z  RotationAngle=0.0  RotationArbitraryAxis=[0 0 1]  FollAlignAxisA=+X  BaseAlignAxisA=+Y  FollAlignAxisB=+Z  BaseAlignAxisB=-X  RotationSequenceAxes=FollowerAxes  RotationSequence=XYX  RotationSequenceAngles=[0 0 0]  RotationSequenceAnglesUnits=deg  RotationMatrix=[1 0 0; 0 1 0; 0 0 1]
  To center : sm_lib/Frames and Transforms/Rigid Transform  TranslationMethod=Cartesian  TranslationStandardOffset=0  TranslationLengthUnit=m  TranslationStandardAxis=+Z  TranslationCartesianOffset=[-thighLength/2 0 0]  TranslationROffset=0  TranslationROffsetUnits=m  TranslationZOffset=0  TranslationZOffsetUnits=m  TranslationThetaOffset=0  TranslationThetaOffsetUnits=deg  RotationMethod=AlignedAxes  RotationAngleUnits=deg  RotationStandardAxis=+Z  RotationAngle=0.0  RotationArbitraryAxis=[0 0 1]  FollAlignAxisA=+Z  BaseAlignAxisA=-X  FollAlignAxisB=+Y  BaseAlignAxisB=+Y  RotationSequenceAxes=FollowerAxes  RotationSequence=XYX  RotationSequenceAngles=[0 0 0]  RotationSequenceAnglesUnits=deg  RotationMatrix=[1 0 0; 0 1 0; 0 0 1]
  knee : PMIOPort  Side=Right
  sensor sheet : PMIOPort  Port=2  Side=Left
  connections:
  To center/RConn1 -- Cylindrical Solid/RConn1
  sensor sheet/RConn1 -- Knee to Sensorsheet/RConn1
  To CG/RConn1 -- Inertia/RConn1
  To center/LConn1 -- knee/RConn1 -- Knee to Sensorsheet/LConn1 -- To CG/LConn1

== system NeuroMuscularLibrary/Thigh total ==
  Leg Load : $bdroot/Leg Load  SystemSampleTime=-1
  Position Sensor : $bdroot/Position Sensor  SystemSampleTime=-1
  Thigh Sensor Sheet : $bdroot/Thigh Sensor Sheet  SystemSampleTime=-1
  Thigh high : $bdroot/Thigh high  thighLength=thighLength  thighMass=thighMass  thighInertiaHigh=thighInertiaHigh  thighKneeToCG=thighKneeToCG
  Thigh low : $bdroot/Thigh low  thighLength=thighLength  thighMass=thighMass  thighInertiaLow=thighInertiaLow  thighKneeToCG=thighKneeToCG
  Velocity Sensor : $bdroot/Velocity Sensor  SystemSampleTime=-1
  Hip : PMIOPort  Side=Right
  Knee : PMIOPort  Port=2  Side=Left
  Leg load : Outport  VectorParamsAs1DForOutWhenUnconnected=on
  Position : Outport  Port=2  VectorParamsAs1DForOutWhenUnconnected=on
  Velocity : Outport  Port=3  VectorParamsAs1DForOutWhenUnconnected=on
  wires:
  Thigh Sensor Sheet/1 -> Leg Load/1
  Leg Load/1 -> Leg load/1
  Position Sensor/1 -> Position/1
  Velocity Sensor/1 -> Velocity/1
  connections:
  Thigh high/LConn1 -- Hip/RConn1
  Knee/RConn1 -- Thigh low/RConn1
  Thigh high/RConn1 -- Position Sensor/LConn1 -- Velocity Sensor/LConn1 -- Thigh Sensor Sheet/RConn1
  Thigh Sensor Sheet/LConn1 -- Thigh low/LConn1

== system NeuroMuscularLibrary/Unit vector ==
  Add : Sum  Inputs=+
  Math Function : Math  Operator=magnitude^2  SaturateOnIntegerOverflow=on
  Position Sensor : $bdroot/Position Sensor  SystemSampleTime=-1
  Product : Product
  Square Root : Sqrt  SaturateOnIntegerOverflow=on
  Frame : PMIOPort  Side=Left
  Unit vector : Outport  VectorParamsAs1DForOutWhenUnconnected=on
  wires:
  Math Function/1 -> Add/1
  Product/1 -> Unit vector/1
  Add/1 -> Square Root/1
  Square Root/1 -> Product/2
  Position Sensor/1 -> Product/1, Math Function/1
  connections:
  Position Sensor/LConn1 -- Frame/RConn1

== system NeuroMuscularLibrary/VAS Link ==
  note: VAS Attachment
  Knee angle [rad] : Inport
  Constant : Constant  Value=lslackVAS+loptVAS
  Constant1 : Constant  Value=phimaxVAS
  Constant2 : Constant  Value=phirefVAS
  Demux : Demux  Outputs=2
  Gain1 : Gain  Gain=rVASmax
  Gain3 : Gain  Gain=phiScaleVAS
  Gain4 : Gain  Gain=rhoVAS/phiScaleVAS
  Gain5 : Gain  Gain=phiScaleVAS
  Mux : Mux  Inputs=2
  Sum1 : Sum  Inputs=-+
  Sum2 : Sum  Inputs=|+-
  Sum3 : Sum  Inputs=-+|
  Sum5 : Sum  Inputs=|++
  length change term : Trigonometry
  offset correction term : Trigonometry
  variable lever term : Trigonometry  Operator=cos
  lmtu [m] : Outport  VectorParamsAs1DForOutWhenUnconnected=on
  lever [m] : Outport  Port=2  VectorParamsAs1DForOutWhenUnconnected=on
  wires:
  Sum1/1 -> Mux/1
  Sum5/1 -> lmtu [m]/1
  offset correction term/1 -> Sum1/1
  Sum2/1 -> Gain5/1
  Constant1/1 -> Sum3/1, Sum2/2
  Constant/1 -> Sum5/1
  Gain3/1 -> variable lever term/1, length change term/1
  Gain1/1 -> Demux/1
  length change term/1 -> Sum1/2
  Constant2/1 -> Sum2/1
  Mux/1 -> Gain1/1
  Gain4/1 -> Sum5/2
  Demux/2 -> lever [m]/1
  variable lever term/1 -> Mux/2
  Sum3/1 -> Gain3/1
  Gain5/1 -> offset correction term/1
  Knee angle [rad]/1 -> Sum3/2
  Demux/1 -> Gain4/1

== system NeuroMuscularLibrary/Velocity Sensor ==
  Mux : Mux  Inputs=3
  PS-Simulink Converter : nesl_utility/PS-Simulink Converter  PhysicalDomain=network_engine_domain  SubClassName=ps_output  LeftPortType=input  RightPortType=output  PseudoPeriodic=off  Frequencies=[]  Unit=m/s  AffineConversion=off
  PS-Simulink Converter1 : nesl_utility/PS-Simulink Converter  PhysicalDomain=network_engine_domain  SubClassName=ps_output  LeftPortType=input  RightPortType=output  PseudoPeriodic=off  Frequencies=[]  Unit=m/s  AffineConversion=off
  PS-Simulink Converter2 : nesl_utility/PS-Simulink Converter  PhysicalDomain=network_engine_domain  SubClassName=ps_output  LeftPortType=input  RightPortType=output  PseudoPeriodic=off  Frequencies=[]  Unit=m/s  AffineConversion=off
  Position Sensor : sm_lib/Frames and Transforms/Transform Sensor  MeasurementFrame=World  SenseAngle=off  SenseAxis=off  SenseAngle1=off  SenseAngle2=off  SenseAngle3=off  SenseQ=off  SenseR=off  SenseOmegaX=off  SenseOmegaY=off  SenseOmegaZ=off  SenseOmega1=off  SenseOmega2=off  SenseOmega3=off  SenseQDot=off  SenseRDot=off  SenseAlphaX=off  SenseAlphaY=off  SenseAlphaZ=off  SenseAlpha1=off  SenseAlpha2=off  SenseAlpha3=off  SenseQDDot=off  SenseRDDot=off  SenseX=off  SenseY=off  SenseZ=off  SenseRad=off  SenseAzim=off  SenseDist=off  SenseInc=off  SenseXDot=on  SenseYDot=on  SenseZDot=on  SenseRadDot=off  SenseAzimDot=off  SenseDistDot=off  SenseIncDot=off  SenseXDDot=off  SenseYDDot=off  SenseZDDot=off  SenseRadDDot=off  SenseAzimDDot=off  SenseDistDDot=off  SenseIncDDot=off
  World Frame : sm_lib/Frames and Transforms/World Frame
  Frame : PMIOPort  Side=Left
  Velocity : Outport  VectorParamsAs1DForOutWhenUnconnected=on
  wires:
  PS-Simulink Converter1/1 -> Mux/2
  PS-Simulink Converter/1 -> Mux/1
  Mux/1 -> Velocity/1
  PS-Simulink Converter2/1 -> Mux/3
  connections:
  Position Sensor/LConn1 -- World Frame/RConn1
  Position Sensor/RConn3 -- PS-Simulink Converter1/LConn1
  Position Sensor/RConn1 -- Frame/RConn1
  Position Sensor/RConn2 -- PS-Simulink Converter/LConn1
  Position Sensor/RConn4 -- PS-Simulink Converter2/LConn1

== system NeuroMuscularLibrary/body pitch//roll//yaw in body frame --- x-axis: forward y-axis: leftward z-axis: parallel to gravity ==
  Left Hip Pos Vel : Inport
  HAT Pos Vel : Inport  Port=2
  Right Hip Pos Vel : Inport  Port=3
  Abs : Abs
  Abs1 : Abs
  Add : Sum  Inputs=+-
  Add1 : Sum  Inputs=-+
  Add2 : Sum  Inputs=+-
  Constant : Constant  Value=2*pi
  Delay One Step : Delay  DelayLength=1
  "Dx, Dy" : Selector  InputPortWidth=3  IndexOptions=Index vector (dialog)  Indices=[1 2]  OutputSizes=1
  "Dx, Dz" : Selector  InputPortWidth=3  IndexOptions=Index vector (dialog)  Indices=[1 2]  OutputSizes=1
  "Dx, Dz1" : Selector  InputPortWidth=3  IndexOptions=Index vector (dialog)  Indices=[1 2]  OutputSizes=1
  "Dz, Dy" : Selector  InputPortWidth=3  IndexOptions=Index vector (dialog)  Indices=[3 2]  OutputSizes=1
  Mean Hip Position and Vel : Gain  Gain=1/2
  Mux{,1..4} (5 alike) : Mux  Inputs=2
  Relational Operator : RelationalOperator  Operator=<=  OutDataTypeStr=boolean  RndMeth=Simplest
  Selector1 : Selector  InputPortWidth=6  IndexOptions=Index vector (dialog)  Indices=[1 2 3]  OutputSizes=1
  Selector3 : Selector  InputPortWidth=6  IndexOptions=Index vector (dialog)  Indices=[1 2 3]  OutputSizes=1
  Selector5 : Selector  InputPortWidth=6  IndexOptions=Index vector (dialog)  Indices=[4 5 6]  OutputSizes=1
  Selector6 : Selector  InputPortWidth=6  IndexOptions=Index vector (dialog)  Indices=[1 2 3]  OutputSizes=1
  Sum1 : Sum
  Sum2 : Sum  Inputs=-+
  Switch : Switch  Criteria=u2 > Threshold
  Theta : Fcn  Expr=atan2(u(1),u(2))
  Theta1 : Fcn  Expr=atan2(u(1),u(2))
  "dDx, dDy" : Selector  InputPortWidth=3  IndexOptions=Index vector (dialog)  Indices=[1 2]  OutputSizes=1
  "dDz, dDy" : Selector  InputPortWidth=3  IndexOptions=Index vector (dialog)  Indices=[3 2]  OutputSizes=1
  dTheta : Fcn  Expr=( u(2)*u(3) - u(1)*u(4) ) / hatLeftHipToCG^2
  dTheta1 : Fcn  Expr=( u(2)*u(3) - u(1)*u(4) ) / hatLeftHipToCG^2
  map1 : Subsystem
  map2 : Subsystem
  new_bases : Subsystem
  yaw1 : Fcn  Expr=pi - atan2(-u(1)+u(3),-u(2)+u(4))
  "pitch, pitch velocity" : Outport  VectorParamsAs1DForOutWhenUnconnected=on
  "roll, roll velocity" : Outport  Port=2  VectorParamsAs1DForOutWhenUnconnected=on
  yaw : Outport  Port=3  VectorParamsAs1DForOutWhenUnconnected=on
  wires:
  "dDx, dDy"/1 -> Mux2/2
  Mux2/1 -> dTheta/1
  HAT Pos Vel/1 -> Sum2/2
  "Dx, Dy"/1 -> Mux2/1, Theta/1
  Selector3/1 -> "Dx, Dz"/1, new_bases/1(L)
  Selector1/1 -> "Dx, Dz1"/1, new_bases/2(R)
  Theta/1 -> Mux/1
  dTheta/1 -> Mux/2
  Selector6/1 -> map1/1(v)
  map1/1(v_new) -> "Dx, Dy"/1, "Dz, Dy"/1
  new_bases/1(bases) -> map1/2(basis), map2/2(basis)
  Selector5/1 -> map2/1(v)
  map2/1(v_new) -> "dDx, dDy"/1, "dDz, dDy"/1
  "dDz, dDy"/1 -> Mux1/2
  Mux1/1 -> dTheta1/1
  "Dz, Dy"/1 -> Mux1/1, Theta1/1
  Theta1/1 -> Mux4/1
  dTheta1/1 -> Mux4/2
  "Dx, Dz"/1 -> Mux3/1
  "Dx, Dz1"/1 -> Mux3/2
  Mux3/1 -> yaw1/1
  yaw1/1 -> Add2/1, Switch/1, Add/1
  Left Hip Pos Vel/1 -> Sum1/1, Selector3/1
  Mean Hip Position and Vel/1 -> Sum2/1
  Sum1/1 -> Mean Hip Position and Vel/1
  Sum2/1 -> Selector6/1, Selector5/1
  Mux/1 -> "pitch, pitch velocity"/1
  Mux4/1 -> "roll, roll velocity"/1
  Right Hip Pos Vel/1 -> Sum1/2, Selector1/1
  Switch/1 -> yaw/1, Delay One Step/1
  Delay One Step/1 -> Add1/1, Add/2
  Add/1 -> Abs/1
  Add1/1 -> Abs1/1
  Abs/1 -> Relational Operator/1
  Abs1/1 -> Relational Operator/2
  Relational Operator/1 -> Switch/2
  Constant/1 -> Add2/2
  Add2/1 -> Switch/3, Add1/2

== system NeuroMuscularLibrary/lateral d, v in body frame ==
  body yaw : Inport
  d0 : Inport  Port=2
  HAT Pos Vel : Inport  Port=3
  Mux1 : Mux  Inputs=2
  Mux2 : Mux  Inputs=2
  Mux3 : Mux  Inputs=2
  Selector1 : Selector  InputPortWidth=3  IndexOptions=Index vector (dialog)  Indices=[1 2]  OutputSizes=1
  Selector2 : Selector  InputPortWidth=6  IndexOptions=Index vector (dialog)  Indices=[1 2 3]  OutputSizes=1
  Selector3 : Selector  InputPortWidth=6  IndexOptions=Index vector (dialog)  Indices=[4 5]  OutputSizes=1
  Sum : Sum  Inputs=-+|
  body frame in transverse plane (xy-plane)1 : Fcn  Expr=u(3)*cos(u(1)) - u(2)*sin(u(1))
  body frame in transverse plane (xy-plane)2 : Fcn  Expr=u(3)*cos(u(1)) - u(2)*sin(u(1))
  body frame in transverse plane (xy-plane)3 : Fcn  Commented=on  Expr=u(2)*sin(u(1)) - u(3)*cos(u(1))
  body frame in transverse plane (xy-plane)4 : Fcn  Commented=on  Expr=u(2)*sin(u(1)) - u(3)*cos(u(1))
  "d, v" : Outport  VectorParamsAs1DForOutWhenUnconnected=on
  wires:
  Sum/1 -> Selector1/1
  Mux1/1 -> body frame in transverse plane (xy-plane)1/1
  body yaw/1 -> Mux2/1, Mux1/1
  Mux2/1 -> body frame in transverse plane (xy-plane)2/1
  d0/1 -> Sum/1
  Selector2/1 -> Sum/2
  body frame in transverse plane (xy-plane)2/1 -> Mux3/2
  Selector3/1 -> Mux2/2
  body frame in transverse plane (xy-plane)1/1 -> Mux3/1
  Mux3/1 -> "d, v"/1
  HAT Pos Vel/1 -> Selector3/1, Selector2/1
  Selector1/1 -> Mux1/2

== system NeuroMuscularLibrary/leg Gait phase detector ==
  StanceSelf : Inport
  StanceOther : Inport  Port=2
  SagPosSelf : Inport  Port=3
  SagPosOther : Inport  Port=4
  normFootShank : Inport  Port=5
  Chart : Stateflow chart  BlockKeywords=__PRM__SERIALIZED__DATA__:Stateflow Chart,Stateflow Diagram  TreatAsAtomicUnit=on
  state : Outport  VectorParamsAs1DForOutWhenUnconnected=on
  wires:
  SagPosOther/1 -> Chart/4(SagPosOther)
  normFootShank/1 -> Chart/5(normFootShank)
  StanceOther/1 -> Chart/2(StanceOther)
  Chart/1(state) -> state/1
  StanceSelf/1 -> Chart/1(StanceSelf)
  SagPosSelf/1 -> Chart/3(SagPosSelf)

== system NeuroMuscularLibrary/sagittal d, v in body frame ==
  body yaw : Inport
  d0 : Inport  Port=2
  HAT Pos Vel : Inport  Port=3
  Mux1 : Mux  Inputs=2
  Mux2 : Mux  Inputs=2
  Mux3 : Mux  Inputs=2
  Selector1 : Selector  InputPortWidth=3  IndexOptions=Index vector (dialog)  Indices=[1 2]  OutputSizes=1
  Selector2 : Selector  InputPortWidth=6  IndexOptions=Index vector (dialog)  Indices=[1 2 3]  OutputSizes=1
  Selector3 : Selector  InputPortWidth=6  IndexOptions=Index vector (dialog)  Indices=[4 5]  OutputSizes=1
  Sum : Sum  Inputs=-+|
  body frame in transverse plane (xz-plane)1 : Fcn  Expr=u(2)*cos(u(1)) - u(3)*sin(u(1))
  body frame in transverse plane (xz-plane)2 : Fcn  Expr=u(2)*cos(u(1)) - u(3)*sin(u(1))
  "d, v" : Outport  VectorParamsAs1DForOutWhenUnconnected=on
  wires:
  Sum/1 -> Selector1/1
  Mux1/1 -> body frame in transverse plane (xz-plane)1/1
  body yaw/1 -> Mux2/1, Mux1/1
  Mux2/1 -> body frame in transverse plane (xz-plane)2/1
  HAT Pos Vel/1 -> Selector3/1, Selector2/1
  body frame in transverse plane (xz-plane)2/1 -> Mux3/2
  Selector3/1 -> Mux2/2
  body frame in transverse plane (xz-plane)1/1 -> Mux3/1
  Mux3/1 -> "d, v"/1
  d0/1 -> Sum/1
  Selector1/1 -> Mux1/2
  Selector2/1 -> Sum/2

== system NeuroMuscularLibrary/Ground Contact Model 3D/3D Contact ==
  RefPt [m m m] : Inport
  nVec [m m m] : Inport  Port=2
  pVec [m m m] : Inport  Port=3
  vVec [m/s m/s m/s] : Inport  Port=4
  Contact! : EnablePort  StatesWhenEnabling=reset
  Friction Switch : Subsystem
  Kinetic Friction Model : Subsystem
  Logical Operator : Logic  Operator=NOT  AllPortsSameDT=off  OutDataTypeStr=boolean
  Static Friction Model : Subsystem
  Sum : Sum
  Sum1 : Sum
  FnVec [N N N] : Outport  OutputWhenDisabled=reset  InitialOutput=[0 0 0]  VectorParamsAs1DForOutWhenUnconnected=on
      settings: AttributesFormatString=when disabled: %<OutputWhenDisabled>
  FtVec [N N N] : Outport  Port=2  OutputWhenDisabled=reset  InitialOutput=[0 0 0]  VectorParamsAs1DForOutWhenUnconnected=on
      settings: AttributesFormatString=when disabled: %<OutputWhenDisabled>
  wires:
  pVec [m m m]/1 -> Static Friction Model/1(pos [m]), Kinetic Friction Model/2(pos [m m m])
  vVec [m/s m/s m/s]/1 -> Kinetic Friction Model/1(vel [m/s m/s m/s]), Static Friction Model/2(vel [m/s m/s m/s])
  Kinetic Friction Model/2(posFP [m m m]) -> Static Friction Model/4(posFP [m])
  Friction Switch/1(Stiction) -> Static Friction Model/Enable, Logical Operator/1
  Logical Operator/1 -> Kinetic Friction Model/Enable
  nVec [m m m]/1 -> Kinetic Friction Model/4(nVec [m m m])
  Kinetic Friction Model/4(Stiction!) -> Friction Switch/2(Stick!)
  Static Friction Model/1(F_n Stick [N N N]) -> Sum1/1
  Kinetic Friction Model/6(F_n Slide [N N N]) -> Sum1/2
  Kinetic Friction Model/5(F_t Slide [N N N]) -> Sum/2
  Static Friction Model/2(F_t Stick [N N N]) -> Sum/1
  Sum1/1 -> FnVec [N N N]/1  "F_nVec"
  Sum/1 -> FtVec [N N N]/1  "F_tVec"
  Static Friction Model/3(Sliding!) -> Friction Switch/1(Slide!)
  RefPt [m m m]/1 -> Kinetic Friction Model/3(RefPt [m m m])
  Kinetic Friction Model/3(nVec FP [m m m]) -> Static Friction Model/5(nVecFP [m m m])
  Kinetic Friction Model/1(RefPtFP [m m m]) -> Static Friction Model/3(RefPtFP [m m m])

== system NeuroMuscularLibrary/Hard Stops/Hip roll Joint Limit ==
  note: Overextension/Overflexion Joint Limit
  phi [rad] : Inport
  dphi [rad/s] : Inport  Port=2
  Gain1 : Gain  Gain=c_jointstop
  Gain2 : Gain  Gain=-1
  Gain3 : Gain  Gain=c_jointstop
  Gain4 : Gain  Gain=1/w_max_jointstop
  Limit Range : simulink/Logic and Bit Operations/Interval Test  Commented=on  IntervalClosedRight=on  uplimit=phi12_UpLimit + 40*pi/180  IntervalClosedLeft=on  lowlimit=phi12_LowLimit - 40*pi/180  OutDataTypeStr=boolean
  Logical Operator3 : Logic  Commented=on  Operator=NOT  AllPortsSameDT=off  OutDataTypeStr=boolean
  Mux1 : Mux  Inputs=2
  Mux3 : Mux  Inputs=2
  Overextension Torque : Fcn  Expr="- u(1)  *  (1-u(2)) * (u(2)<1) * (u(1)>0)"
  Overflexion Torque : Fcn  Expr="- u(1)  *  (1-u(2)) * (u(2)<1) * (u(1)<0)"
  Stop Simulation1 : Stop  Commented=on
  Sum : Sum  Inputs=|+-
  Sum1 : Sum  Inputs=|+-
  Sum2 : Sum
  overextension angle : Constant  Value=phiUpLimit
  overflexion angle : Constant  Value=phiLowLimit
  M_stop [Nm] : Outport  VectorParamsAs1DForOutWhenUnconnected=on
  wires:
  Mux3/1 -> Overextension Torque/1
  Gain3/1 -> Mux3/1
  dphi [rad/s]/1 -> Gain4/1
  overextension angle/1 -> Sum/2
  phi [rad]/1 -> Sum/1, Sum1/1, Limit Range/1
  Sum/1 -> Gain3/1
  Gain4/1 -> Gain2/1, Mux1/2
  Gain1/1 -> Mux1/1
  Sum1/1 -> Gain1/1
  overflexion angle/1 -> Sum1/2
  Mux1/1 -> Overflexion Torque/1
  Sum2/1 -> M_stop [Nm]/1
  Gain2/1 -> Mux3/2
  Overflexion Torque/1 -> Sum2/2
  Overextension Torque/1 -> Sum2/1
  Limit Range/1 -> Logical Operator3/1
  Logical Operator3/1 -> Stop Simulation1/1

== system NeuroMuscularLibrary/Hill Muscle/BE force-length relation ==
  note: Buffer Elasticity BE
  lce [lopt] : Inport
  Constant1 : Constant  Value=1-w
  Math Function : Math  Operator=square  SaturateOnIntegerOverflow=on
  Mux1 : Mux  Inputs=2
  Sum4 : Sum  Inputs=|+-  SaturateOnIntegerOverflow=on  InputSameDT=on  OutDataTypeStr=Inherit: Same as first input
  force above slack length : Fcn  Expr=u(2)*(u(1)<0)
  reference strain [lslack] : Constant  Value=w/2
  relative strain : Product  Inputs=*/
  fbe [Fmax] : Outport  VectorParamsAs1DForOutWhenUnconnected=on
  wires:
  Constant1/1 -> Sum4/2
  Sum4/1 -> Mux1/1, relative strain/1
  reference strain [lslack]/1 -> relative strain/2
  relative strain/1 -> Math Function/1
  Math Function/1 -> Mux1/2
  force above slack length/1 -> fbe [Fmax]/1
  Mux1/1 -> force above slack length/1
  lce [lopt]/1 -> Sum4/1
